simulink model "test_mdl"  (R2018a)
settings: Solver=VariableStepAuto  StartTime=0.0  StopTime=10.0  RelTol=1e-3
(part 3 of 8)

== system test_mdl/FD1_CAN_P702_GASD_MY21_DCV_V06/GWM/AC_Compressor_Data_FD1 ==
  ElCmprBattSysU_D_Falt : Constant
  ElCmprBattURng_D_Falt : Constant
  ElCmprInnrErr_D_Falt : Constant
  ElCmprLostComm_D_Falt : Constant
  ElCmprOverLoad_D_Falt : Constant
  ElCmprOverTe_D_Falt : Constant
  ElCmprOverTe_D_Stat : Constant
  ElCmprPerfErr_D_Falt : Constant
  ElCmprSysU_D_Falt : Constant
  ElCmprUHi_D_Stat : Constant
  ElCmprUHi_U_Actl : Constant
  ElCmpr_D_Stat : Constant
  ElCmpr_N_Actl : Constant
  ElCmpr_Pw_Actl : Constant
  bus_creator : BusCreator  Inputs=14
  port : Outport
  wires:
  bus_creator/1 -> port/1  "AC_Compressor_Data_FD1"
  ElCmprBattSysU_D_Falt/1 -> bus_creator/1  "ElCmprBattSysU_D_Falt"
  ElCmprBattURng_D_Falt/1 -> bus_creator/2  "ElCmprBattURng_D_Falt"
  ElCmprInnrErr_D_Falt/1 -> bus_creator/3  "ElCmprInnrErr_D_Falt"
  ElCmprLostComm_D_Falt/1 -> bus_creator/4  "ElCmprLostComm_D_Falt"
  ElCmprOverLoad_D_Falt/1 -> bus_creator/5  "ElCmprOverLoad_D_Falt"
  ElCmprOverTe_D_Falt/1 -> bus_creator/6  "ElCmprOverTe_D_Falt"
  ElCmprOverTe_D_Stat/1 -> bus_creator/7  "ElCmprOverTe_D_Stat"
  ElCmprPerfErr_D_Falt/1 -> bus_creator/8  "ElCmprPerfErr_D_Falt"
  ElCmprSysU_D_Falt/1 -> bus_creator/9  "ElCmprSysU_D_Falt"
  ElCmprUHi_D_Stat/1 -> bus_creator/10  "ElCmprUHi_D_Stat"
  ElCmprUHi_U_Actl/1 -> bus_creator/11  "ElCmprUHi_U_Actl"
  ElCmpr_D_Stat/1 -> bus_creator/12  "ElCmpr_D_Stat"
  ElCmpr_N_Actl/1 -> bus_creator/13  "ElCmpr_N_Actl"
  ElCmpr_Pw_Actl/1 -> bus_creator/14  "ElCmpr_Pw_Actl"

== system test_mdl/FD1_CAN_P702_GASD_MY21_DCV_V06/GWM/APIMGPS_Data_Nav_1_FD1 ==
  GPS_Latitude_Degrees : Constant
  GPS_Latitude_Min_dec : Constant
  GPS_Latitude_Minutes : Constant
  GPS_Longitude_Degrees : Constant
  GPS_Longitude_Min_dec : Constant
  GPS_Longitude_Minutes : Constant
  GpsHsphLattSth_D_Actl : Constant
  GpsHsphLongEast_D_Actl : Constant
  bus_creator : BusCreator  Inputs=8
  port : Outport
  wires:
  bus_creator/1 -> port/1  "APIMGPS_Data_Nav_1_FD1"
  GPS_Latitude_Degrees/1 -> bus_creator/1  "GPS_Latitude_Degrees"
  GPS_Latitude_Min_dec/1 -> bus_creator/2  "GPS_Latitude_Min_dec"
  GPS_Latitude_Minutes/1 -> bus_creator/3  "GPS_Latitude_Minutes"
  GPS_Longitude_Degrees/1 -> bus_creator/4  "GPS_Longitude_Degrees"
  GPS_Longitude_Min_dec/1 -> bus_creator/5  "GPS_Longitude_Min_dec"
  GPS_Longitude_Minutes/1 -> bus_creator/6  "GPS_Longitude_Minutes"
  GpsHsphLattSth_D_Actl/1 -> bus_creator/7  "GpsHsphLattSth_D_Actl"
  GpsHsphLongEast_D_Actl/1 -> bus_creator/8  "GpsHsphLongEast_D_Actl"

== system test_mdl/FD1_CAN_P702_GASD_MY21_DCV_V06/GWM/APIMGPS_Data_Nav_2_FD1 ==
  GPS_Actual_vs_Infer_pos : Constant
  GPS_Compass_direction : Constant
  GPS_Pdop : Constant
  GPS_UTC_hours : Constant
  GPS_UTC_minutes : Constant
  GPS_UTC_seconds : Constant
  GpsUtcDay_No_Actl : Constant
  GpsUtcMnth_No_Actl : Constant
  GpsUtcYr_No_Actl : Constant
  Gps_B_Falt : Constant
  bus_creator : BusCreator  Inputs=10
  port : Outport
  wires:
  bus_creator/1 -> port/1  "APIMGPS_Data_Nav_2_FD1"
  GPS_Actual_vs_Infer_pos/1 -> bus_creator/1  "GPS_Actual_vs_Infer_pos"
  GPS_Compass_direction/1 -> bus_creator/2  "GPS_Compass_direction"
  GPS_Pdop/1 -> bus_creator/3  "GPS_Pdop"
  GPS_UTC_hours/1 -> bus_creator/4  "GPS_UTC_hours"
  GPS_UTC_minutes/1 -> bus_creator/5  "GPS_UTC_minutes"
  GPS_UTC_seconds/1 -> bus_creator/6  "GPS_UTC_seconds"
  GpsUtcDay_No_Actl/1 -> bus_creator/7  "GpsUtcDay_No_Actl"
  GpsUtcMnth_No_Actl/1 -> bus_creator/8  "GpsUtcMnth_No_Actl"
  GpsUtcYr_No_Actl/1 -> bus_creator/9  "GpsUtcYr_No_Actl"
  Gps_B_Falt/1 -> bus_creator/10  "Gps_B_Falt"

== system test_mdl/FD1_CAN_P702_GASD_MY21_DCV_V06/GWM/APIMGPS_Data_Nav_3_FD1 ==
  GPS_Hdop : Constant
  GPS_Heading : Constant
  GPS_MSL_altitude : Constant
  GPS_Sat_num_in_view : Constant
  GPS_Speed : Constant
  GPS_Vdop : Constant
  GPS_dimension : Constant
  bus_creator : BusCreator  Inputs=7
  port : Outport
  wires:
  bus_creator/1 -> port/1  "APIMGPS_Data_Nav_3_FD1"
  GPS_Hdop/1 -> bus_creator/1  "GPS_Hdop"
  GPS_Heading/1 -> bus_creator/2  "GPS_Heading"
  GPS_MSL_altitude/1 -> bus_creator/3  "GPS_MSL_altitude"
  GPS_Sat_num_in_view/1 -> bus_creator/4  "GPS_Sat_num_in_view"
  GPS_Speed/1 -> bus_creator/5  "GPS_Speed"
  GPS_Vdop/1 -> bus_creator/6  "GPS_Vdop"
  GPS_dimension/1 -> bus_creator/7  "GPS_dimension"

== system test_mdl/FD1_CAN_P702_GASD_MY21_DCV_V06/GWM/APIM_Data_FD1 ==
  AutoLghtOvrrd_B_RqDrv : Constant
  DistToStopover_L_Actl : Constant
  ExtLghtDsply_D_Stat : Constant
  ExtLghtFront_D_RqMnu : Constant
  ExtLghtLeft_D_RqMnu : Constant
  ExtLghtRear_D_RqMnu : Constant
  ExtLghtRight_D_RqMnu : Constant
  GoTEditHr_T_RqMnu : Constant
  GoTEditMnte_T_RqMnu : Constant
  StopoverType_D_Stat : Constant
  bus_creator : BusCreator  Inputs=10
  port : Outport
  wires:
  bus_creator/1 -> port/1  "APIM_Data_FD1"
  AutoLghtOvrrd_B_RqDrv/1 -> bus_creator/1  "AutoLghtOvrrd_B_RqDrv"
  DistToStopover_L_Actl/1 -> bus_creator/2  "DistToStopover_L_Actl"
  ExtLghtDsply_D_Stat/1 -> bus_creator/3  "ExtLghtDsply_D_Stat"
  ExtLghtFront_D_RqMnu/1 -> bus_creator/4  "ExtLghtFront_D_RqMnu"
  ExtLghtLeft_D_RqMnu/1 -> bus_creator/5  "ExtLghtLeft_D_RqMnu"
  ExtLghtRear_D_RqMnu/1 -> bus_creator/6  "ExtLghtRear_D_RqMnu"
  ExtLghtRight_D_RqMnu/1 -> bus_creator/7  "ExtLghtRight_D_RqMnu"
  GoTEditHr_T_RqMnu/1 -> bus_creator/8  "GoTEditHr_T_RqMnu"
  GoTEditMnte_T_RqMnu/1 -> bus_creator/9  "GoTEditMnte_T_RqMnu"
  StopoverType_D_Stat/1 -> bus_creator/10  "StopoverType_D_Stat"

== system test_mdl/FD1_CAN_P702_GASD_MY21_DCV_V06/GWM/APIM_Request_Signals_1_FD1 ==
  Btt_L_Actl2 : Constant
  ChrgCrdLckEnbl_B_Stat : Constant
  ChrgOvrdExitScrn_D_Rq : Constant
  Cntr_Plg_Mode_Cmd : Constant
  EmPrflButtnAssoc_D_Rq : Constant
  EmPrflKeyAssoc_D_Rq : Constant
  EmPrflNo_D_Rq : Constant
  Em_D_Stat : Constant
  PmCabnLvl_D_Stat : Constant
  PmCabn_D_Stat : Constant
  PwRnngBoardMde_D_Rq : Constant
  PwRnngBoardSwtch_D_Rq : Constant
  PwRnngBoardT_D_Rq : Constant
  Rba_D_Rq : Constant
  bus_creator : BusCreator  Inputs=14
  port : Outport
  wires:
  bus_creator/1 -> port/1  "APIM_Request_Signals_1_FD1"
  Btt_L_Actl2/1 -> bus_creator/1  "Btt_L_Actl2"
  ChrgCrdLckEnbl_B_Stat/1 -> bus_creator/2  "ChrgCrdLckEnbl_B_Stat"
  ChrgOvrdExitScrn_D_Rq/1 -> bus_creator/3  "ChrgOvrdExitScrn_D_Rq"
  Cntr_Plg_Mode_Cmd/1 -> bus_creator/4  "Cntr_Plg_Mode_Cmd"
  EmPrflButtnAssoc_D_Rq/1 -> bus_creator/5  "EmPrflButtnAssoc_D_Rq"
  EmPrflKeyAssoc_D_Rq/1 -> bus_creator/6  "EmPrflKeyAssoc_D_Rq"
  EmPrflNo_D_Rq/1 -> bus_creator/7  "EmPrflNo_D_Rq"
  Em_D_Stat/1 -> bus_creator/8  "Em_D_Stat"
  PmCabnLvl_D_Stat/1 -> bus_creator/9  "PmCabnLvl_D_Stat"
  PmCabn_D_Stat/1 -> bus_creator/10  "PmCabn_D_Stat"
  PwRnngBoardMde_D_Rq/1 -> bus_creator/11  "PwRnngBoardMde_D_Rq"
  PwRnngBoardSwtch_D_Rq/1 -> bus_creator/12  "PwRnngBoardSwtch_D_Rq"
  PwRnngBoardT_D_Rq/1 -> bus_creator/13  "PwRnngBoardT_D_Rq"
  Rba_D_Rq/1 -> bus_creator/14  "Rba_D_Rq"

== system test_mdl/FD1_CAN_P702_GASD_MY21_DCV_V06/GWM/APIM_Request_Signals_5_FD1 ==
  OnbChrgLocIdTrgt_No_Rq : Constant
  OnbChrgLocIdUns_B_Rq : Constant
  OnbChrgPrflUpdate_B_Rq : Constant
  OnbChrgPrflWkdy_No_Rq : Constant
  OnbChrgPrflWknd_No_Rq : Constant
  OnbChrgSetDelete_B_Rq : Constant
  OnbChrgSetNow_D_Rq : Constant
  OnbChrgToPcWkdy_D_Actl : Constant
  OnbChrgToPcWknd_D_Actl : Constant
  bus_creator : BusCreator  Inputs=9
  port : Outport
  wires:
  bus_creator/1 -> port/1  "APIM_Request_Signals_5_FD1"
  OnbChrgLocIdTrgt_No_Rq/1 -> bus_creator/1  "OnbChrgLocIdTrgt_No_Rq"
  OnbChrgLocIdUns_B_Rq/1 -> bus_creator/2  "OnbChrgLocIdUns_B_Rq"
  OnbChrgPrflUpdate_B_Rq/1 -> bus_creator/3  "OnbChrgPrflUpdate_B_Rq"
  OnbChrgPrflWkdy_No_Rq/1 -> bus_creator/4  "OnbChrgPrflWkdy_No_Rq"
  OnbChrgPrflWknd_No_Rq/1 -> bus_creator/5  "OnbChrgPrflWknd_No_Rq"
  OnbChrgSetDelete_B_Rq/1 -> bus_creator/6  "OnbChrgSetDelete_B_Rq"
  OnbChrgSetNow_D_Rq/1 -> bus_creator/7  "OnbChrgSetNow_D_Rq"
  OnbChrgToPcWkdy_D_Actl/1 -> bus_creator/8  "OnbChrgToPcWkdy_D_Actl"
  OnbChrgToPcWknd_D_Actl/1 -> bus_creator/9  "OnbChrgToPcWknd_D_Actl"

== system test_mdl/FD1_CAN_P702_GASD_MY21_DCV_V06/GWM/APIM_Request_Signals_FD1 ==
  CbnCmrtPrefListIndx_Rq : Constant
  CbnCmrtPrefLstNmItm_Rq : Constant
  ChrgStatDsply_D_Rq : Constant
  FactoryReset_Rq : Constant
  LongTermParking_Rq : Constant
  ModemReset_D_Rq : Constant
  NextUsageTimeToggle_Rq : Constant
  OffPeakTimeSetHR_Rq : Constant
  OffPeakTimeSetMin_Rq : Constant
  StopStrtDrvMde_B_RqBtn3 : Constant
  TCU_ESN_D_Rq : Constant
  bus_creator : BusCreator  Inputs=11
  port : Outport
  wires:
  bus_creator/1 -> port/1  "APIM_Request_Signals_FD1"
  CbnCmrtPrefListIndx_Rq/1 -> bus_creator/1  "CbnCmrtPrefListIndx_Rq"
  CbnCmrtPrefLstNmItm_Rq/1 -> bus_creator/2  "CbnCmrtPrefLstNmItm_Rq"
  ChrgStatDsply_D_Rq/1 -> bus_creator/3  "ChrgStatDsply_D_Rq"
  FactoryReset_Rq/1 -> bus_creator/4  "FactoryReset_Rq"
  LongTermParking_Rq/1 -> bus_creator/5  "LongTermParking_Rq"
  ModemReset_D_Rq/1 -> bus_creator/6  "ModemReset_D_Rq"
  NextUsageTimeToggle_Rq/1 -> bus_creator/7  "NextUsageTimeToggle_Rq"
  OffPeakTimeSetHR_Rq/1 -> bus_creator/8  "OffPeakTimeSetHR_Rq"
  OffPeakTimeSetMin_Rq/1 -> bus_creator/9  "OffPeakTimeSetMin_Rq"
  StopStrtDrvMde_B_RqBtn3/1 -> bus_creator/10  "StopStrtDrvMde_B_RqBtn3"
  TCU_ESN_D_Rq/1 -> bus_creator/11  "TCU_ESN_D_Rq"

== system test_mdl/FD1_CAN_P702_GASD_MY21_DCV_V06/GWM/APIM_Send_Signals1_FD1 ==
  APIM_ActiveTrackNum_St : Constant
  APIM_NumberofTracks_St : Constant
  AutoHoldSwtch_D_Stat3 : Constant
  CenterStackRing_D_Actl : Constant
  ChrgCordUnlock_B_Rq : Constant
  TrlrAidCancl_B_Rq : Constant
  TrlrAidSetup_D_Stat : Constant
  TrlrTrgtAcquire_D_Rq : Constant
  ValetMode_D_Stat : Constant
  bus_creator : BusCreator  Inputs=9
  port : Outport
  wires:
  bus_creator/1 -> port/1  "APIM_Send_Signals1_FD1"
  APIM_ActiveTrackNum_St/1 -> bus_creator/1  "APIM_ActiveTrackNum_St"
  APIM_NumberofTracks_St/1 -> bus_creator/2  "APIM_NumberofTracks_St"
  AutoHoldSwtch_D_Stat3/1 -> bus_creator/3  "AutoHoldSwtch_D_Stat3"
  CenterStackRing_D_Actl/1 -> bus_creator/4  "CenterStackRing_D_Actl"
  ChrgCordUnlock_B_Rq/1 -> bus_creator/5  "ChrgCordUnlock_B_Rq"
  TrlrAidCancl_B_Rq/1 -> bus_creator/6  "TrlrAidCancl_B_Rq"
  TrlrAidSetup_D_Stat/1 -> bus_creator/7  "TrlrAidSetup_D_Stat"
  TrlrTrgtAcquire_D_Rq/1 -> bus_creator/8  "TrlrTrgtAcquire_D_Rq"
  ValetMode_D_Stat/1 -> bus_creator/9  "ValetMode_D_Stat"

== system test_mdl/FD1_CAN_P702_GASD_MY21_DCV_V06/GWM/APIM_Send_Signals_2_FD1 ==
  AutoEpbButtn_B_Stat : Constant
  AutoEpbZoomView_B_Stat : Constant
  DcacGfciTestBttn_B_Stat : Constant
  DcacPwButtn_B_Falt : Constant
  DcacPwHiButtn_B_Stat : Constant
  DcacPwLoButtn_B_Stat : Constant
  DcacPwOffButtn_B_Stat : Constant
  DcacPwResetButtn_B_Stat : Constant
  OnbChrgClearAll_B_Rq : Constant
  OnbChrgGoTDelete_B_Rq : Constant
  OnbChrgGoTElement_D_Rq : Constant
  OnbChrgGoTExtHtr_D_Rq : Constant
  OnbChrgGoTHr_T_Rq : Constant
  OnbChrgGoTMnte_D_Rq : Constant
  OnbChrgGoTOn_D_Rq : Constant
  OnbChrgGoTPrcond_D_Rq : Constant
  OnbChrgGoTTouch_D_Rq : Constant
  OnbChrgGoTUpdate_B_Rq : Constant
  OtaTrg_D_Stat : Constant
  PaakMyKey_D_Rq : Constant
  TCU_Final_Actvtn_St : Constant
  TCU_Init_Actvtn_St : Constant
  TrlrAidMde_D_Rq : Constant
  TrlrBrkGain_No_Rq : Constant
  TrlrHitch_D_RqMnu : Constant
  bus_creator : BusCreator  Inputs=25
  port : Outport
  wires:
  bus_creator/1 -> port/1  "APIM_Send_Signals_2_FD1"
  AutoEpbButtn_B_Stat/1 -> bus_creator/1  "AutoEpbButtn_B_Stat"
  AutoEpbZoomView_B_Stat/1 -> bus_creator/2  "AutoEpbZoomView_B_Stat"
  DcacGfciTestBttn_B_Stat/1 -> bus_creator/3  "DcacGfciTestBttn_B_Stat"
  DcacPwButtn_B_Falt/1 -> bus_creator/4  "DcacPwButtn_B_Falt"
  DcacPwHiButtn_B_Stat/1 -> bus_creator/5  "DcacPwHiButtn_B_Stat"
  DcacPwLoButtn_B_Stat/1 -> bus_creator/6  "DcacPwLoButtn_B_Stat"
  DcacPwOffButtn_B_Stat/1 -> bus_creator/7  "DcacPwOffButtn_B_Stat"
  DcacPwResetButtn_B_Stat/1 -> bus_creator/8  "DcacPwResetButtn_B_Stat"
  OnbChrgClearAll_B_Rq/1 -> bus_creator/9  "OnbChrgClearAll_B_Rq"
  OnbChrgGoTDelete_B_Rq/1 -> bus_creator/10  "OnbChrgGoTDelete_B_Rq"
  OnbChrgGoTElement_D_Rq/1 -> bus_creator/11  "OnbChrgGoTElement_D_Rq"
  OnbChrgGoTExtHtr_D_Rq/1 -> bus_creator/12  "OnbChrgGoTExtHtr_D_Rq"
  OnbChrgGoTHr_T_Rq/1 -> bus_creator/13  "OnbChrgGoTHr_T_Rq"
  OnbChrgGoTMnte_D_Rq/1 -> bus_creator/14  "OnbChrgGoTMnte_D_Rq"
  OnbChrgGoTOn_D_Rq/1 -> bus_creator/15  "OnbChrgGoTOn_D_Rq"
  OnbChrgGoTPrcond_D_Rq/1 -> bus_creator/16  "OnbChrgGoTPrcond_D_Rq"
  OnbChrgGoTTouch_D_Rq/1 -> bus_creator/17  "OnbChrgGoTTouch_D_Rq"
  OnbChrgGoTUpdate_B_Rq/1 -> bus_creator/18  "OnbChrgGoTUpdate_B_Rq"
  OtaTrg_D_Stat/1 -> bus_creator/19  "OtaTrg_D_Stat"
  PaakMyKey_D_Rq/1 -> bus_creator/20  "PaakMyKey_D_Rq"
  TCU_Final_Actvtn_St/1 -> bus_creator/21  "TCU_Final_Actvtn_St"
  TCU_Init_Actvtn_St/1 -> bus_creator/22  "TCU_Init_Actvtn_St"
  TrlrAidMde_D_Rq/1 -> bus_creator/23  "TrlrAidMde_D_Rq"
  TrlrBrkGain_No_Rq/1 -> bus_creator/24  "TrlrBrkGain_No_Rq"
  TrlrHitch_D_RqMnu/1 -> bus_creator/25  "TrlrHitch_D_RqMnu"

== system test_mdl/FD1_CAN_P702_GASD_MY21_DCV_V06/GWM/Accel_Data_FD1 ==
  VehLat2_A_Actl : Constant
  VehLatAActl_D_Qf : Constant
  VehLatLongVertA_No_Cs : Constant
  VehLatLongVert_No_Cnt : Constant
  VehLong2_A_Actl : Constant
  VehLongAActl_D_Qf : Constant
  VehVert2_A_Actl : Constant
  VehVertAActl_D_Qf : Constant
  bus_creator : BusCreator  Inputs=8
  port : Outport
  wires:
  bus_creator/1 -> port/1  "Accel_Data_FD1"
  VehLat2_A_Actl/1 -> bus_creator/1  "VehLat2_A_Actl"
  VehLatAActl_D_Qf/1 -> bus_creator/2  "VehLatAActl_D_Qf"
  VehLatLongVertA_No_Cs/1 -> bus_creator/3  "VehLatLongVertA_No_Cs"
  VehLatLongVert_No_Cnt/1 -> bus_creator/4  "VehLatLongVert_No_Cnt"
  VehLong2_A_Actl/1 -> bus_creator/5  "VehLong2_A_Actl"
  VehLongAActl_D_Qf/1 -> bus_creator/6  "VehLongAActl_D_Qf"
  VehVert2_A_Actl/1 -> bus_creator/7  "VehVert2_A_Actl"
  VehVertAActl_D_Qf/1 -> bus_creator/8  "VehVertAActl_D_Qf"

== system test_mdl/FD1_CAN_P702_GASD_MY21_DCV_V06/GWM/ActiveFrontStrg_Stat2_FD1 ==
  SteWhlRelCalib_An_Sns : Constant
  SteWhlRelCalib_T_Actl : Constant
  bus_creator : BusCreator  Inputs=2
  port : Outport
  wires:
  bus_creator/1 -> port/1  "ActiveFrontStrg_Stat2_FD1"
  SteWhlRelCalib_An_Sns/1 -> bus_creator/1  "SteWhlRelCalib_An_Sns"
  SteWhlRelCalib_T_Actl/1 -> bus_creator/2  "SteWhlRelCalib_T_Actl"

== system test_mdl/FD1_CAN_P702_GASD_MY21_DCV_V06/GWM/ActiveFrontStrg_Stat_FD1 ==
  SteWhlBrkAnActl_No_Cnt : Constant
  SteWhlBrkAnActl_No_Cs : Constant
  SteWhlBrkOffst_An_Actl : Constant
  SteWhlOffstRq_D_Stat : Constant
  SteWhlOffst_An_TotActl : Constant
  bus_creator : BusCreator  Inputs=5
  port : Outport
  wires:
  bus_creator/1 -> port/1  "ActiveFrontStrg_Stat_FD1"
  SteWhlBrkAnActl_No_Cnt/1 -> bus_creator/1  "SteWhlBrkAnActl_No_Cnt"
  SteWhlBrkAnActl_No_Cs/1 -> bus_creator/2  "SteWhlBrkAnActl_No_Cs"
  SteWhlBrkOffst_An_Actl/1 -> bus_creator/3  "SteWhlBrkOffst_An_Actl"
  SteWhlOffstRq_D_Stat/1 -> bus_creator/4  "SteWhlOffstRq_D_Stat"
  SteWhlOffst_An_TotActl/1 -> bus_creator/5  "SteWhlOffst_An_TotActl"

== system test_mdl/FD1_CAN_P702_GASD_MY21_DCV_V06/GWM/Adaptive_Headlamp_Stat ==
  Adaptive_Hdlmp_Fault : Constant
  AhbStatGfhbFdbk_D_Actl : Constant
  HeadLghtDrvSide_B_Stat : Constant
  HeadLghtHiOn_B_StatHcm : Constant
  bus_creator : BusCreator  Inputs=4
  port : Outport
  wires:
  bus_creator/1 -> port/1  "Adaptive_Headlamp_Stat"
  Adaptive_Hdlmp_Fault/1 -> bus_creator/1  "Adaptive_Hdlmp_Fault"
  AhbStatGfhbFdbk_D_Actl/1 -> bus_creator/2  "AhbStatGfhbFdbk_D_Actl"
  HeadLghtDrvSide_B_Stat/1 -> bus_creator/3  "HeadLghtDrvSide_B_Stat"
  HeadLghtHiOn_B_StatHcm/1 -> bus_creator/4  "HeadLghtHiOn_B_StatHcm"

== system test_mdl/FD1_CAN_P702_GASD_MY21_DCV_V06/GWM/AllTerrainControlData_FD1 ==
  SelDrvMdeCnt_D_Stat : Constant
  SelDrvMdeSwtch_D_Stat : Constant
  SelDrvMdeSwtch_No_Actl : Constant
  bus_creator : BusCreator  Inputs=3
  port : Outport
  wires:
  bus_creator/1 -> port/1  "AllTerrainControlData_FD1"
  SelDrvMdeCnt_D_Stat/1 -> bus_creator/1  "SelDrvMdeCnt_D_Stat"
  SelDrvMdeSwtch_D_Stat/1 -> bus_creator/2  "SelDrvMdeSwtch_D_Stat"
  SelDrvMdeSwtch_No_Actl/1 -> bus_creator/3  "SelDrvMdeSwtch_No_Actl"

== system test_mdl/FD1_CAN_P702_GASD_MY21_DCV_V06/GWM/All_Terrain_Data_FD1 ==
  TerrMde_D_RqDrv : Constant
  bus_creator : BusCreator  Inputs=1
  port : Outport
  wires:
  bus_creator/1 -> port/1  "All_Terrain_Data_FD1"
  TerrMde_D_RqDrv/1 -> bus_creator/1  "TerrMde_D_RqDrv"

== system test_mdl/FD1_CAN_P702_GASD_MY21_DCV_V06/GWM/BCMC_Data_FD1 ==
  WndwRearHeat_D_Stat : Constant
  WndwRearHeat_I_Actl : Constant
  bus_creator : BusCreator  Inputs=2
  port : Outport
  wires:
  bus_creator/1 -> port/1  "BCMC_Data_FD1"
  WndwRearHeat_D_Stat/1 -> bus_creator/1  "WndwRearHeat_D_Stat"
  WndwRearHeat_I_Actl/1 -> bus_creator/2  "WndwRearHeat_I_Actl"

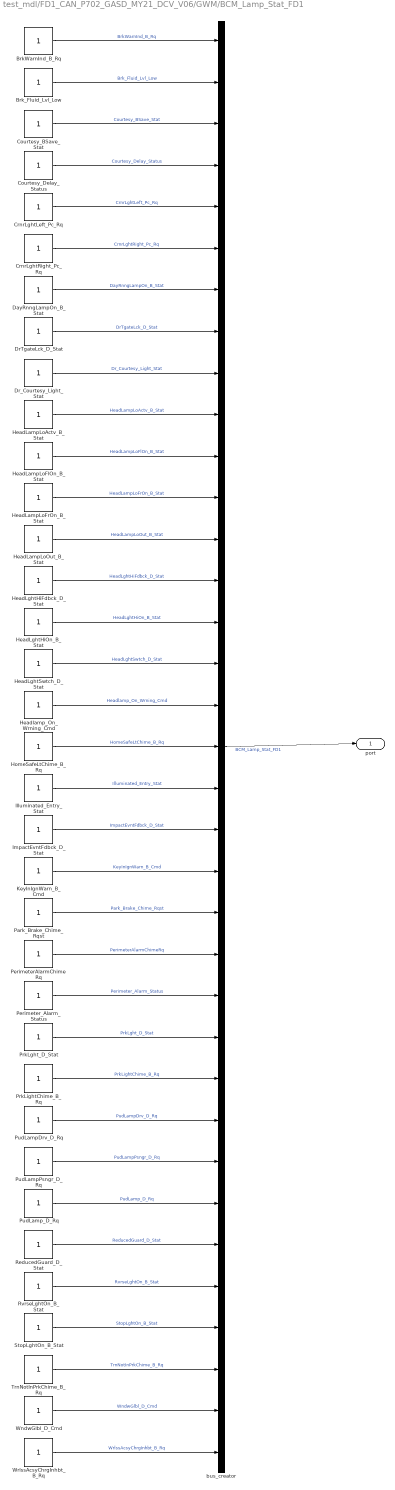
== system test_mdl/FD1_CAN_P702_GASD_MY21_DCV_V06/GWM/BCM_Lamp_Stat_FD1 ==
  BrkWarnInd_B_Rq : Constant
  Brk_Fluid_Lvl_Low : Constant
  Courtesy_BSave_Stat : Constant
  Courtesy_Delay_Status : Constant
  CrnrLghtLeft_Pc_Rq : Constant
  CrnrLghtRight_Pc_Rq : Constant
  DayRnngLampOn_B_Stat : Constant
  DrTgateLck_D_Stat : Constant
  Dr_Courtesy_Light_Stat : Constant
  HeadLampLoActv_B_Stat : Constant
  HeadLampLoFlOn_B_Stat : Constant
  HeadLampLoFrOn_B_Stat : Constant
  HeadLampLoOut_B_Stat : Constant
  HeadLghtHiFdbck_D_Stat : Constant
  HeadLghtHiOn_B_Stat : Constant
  HeadLghtSwtch_D_Stat : Constant
  Headlamp_On_Wrning_Cmd : Constant
  HomeSafeLtChime_B_Rq : Constant
  Illuminated_Entry_Stat : Constant
  ImpactEvntFdbck_D_Stat : Constant
  KeyInIgnWarn_B_Cmd : Constant
  Park_Brake_Chime_Rqst : Constant
  PerimeterAlarmChimeRq : Constant
  Perimeter_Alarm_Status : Constant
  PrkLght_D_Stat : Constant
  PrkLightChime_B_Rq : Constant
  PudLampDrv_D_Rq : Constant
  PudLampPsngr_D_Rq : Constant
  PudLamp_D_Rq : Constant
  ReducedGuard_D_Stat : Constant
  RvrseLghtOn_B_Stat : Constant
  StopLghtOn_B_Stat : Constant
  TrnNotInPrkChime_B_Rq : Constant
  WndwGlbl_D_Cmd : Constant
  WrlssAcsyChrgInhbt_B_Rq : Constant
  bus_creator : BusCreator  Inputs=35
  port : Outport
  wires:
  bus_creator/1 -> port/1  "BCM_Lamp_Stat_FD1"
  BrkWarnInd_B_Rq/1 -> bus_creator/1  "BrkWarnInd_B_Rq"
  Brk_Fluid_Lvl_Low/1 -> bus_creator/2  "Brk_Fluid_Lvl_Low"
  Courtesy_BSave_Stat/1 -> bus_creator/3  "Courtesy_BSave_Stat"
  Courtesy_Delay_Status/1 -> bus_creator/4  "Courtesy_Delay_Status"
  CrnrLghtLeft_Pc_Rq/1 -> bus_creator/5  "CrnrLghtLeft_Pc_Rq"
  CrnrLghtRight_Pc_Rq/1 -> bus_creator/6  "CrnrLghtRight_Pc_Rq"
  DayRnngLampOn_B_Stat/1 -> bus_creator/7  "DayRnngLampOn_B_Stat"
  DrTgateLck_D_Stat/1 -> bus_creator/8  "DrTgateLck_D_Stat"
  Dr_Courtesy_Light_Stat/1 -> bus_creator/9  "Dr_Courtesy_Light_Stat"
  HeadLampLoActv_B_Stat/1 -> bus_creator/10  "HeadLampLoActv_B_Stat"
  HeadLampLoFlOn_B_Stat/1 -> bus_creator/11  "HeadLampLoFlOn_B_Stat"
  HeadLampLoFrOn_B_Stat/1 -> bus_creator/12  "HeadLampLoFrOn_B_Stat"
  HeadLampLoOut_B_Stat/1 -> bus_creator/13  "HeadLampLoOut_B_Stat"
  HeadLghtHiFdbck_D_Stat/1 -> bus_creator/14  "HeadLghtHiFdbck_D_Stat"
  HeadLghtHiOn_B_Stat/1 -> bus_creator/15  "HeadLghtHiOn_B_Stat"
  HeadLghtSwtch_D_Stat/1 -> bus_creator/16  "HeadLghtSwtch_D_Stat"
  Headlamp_On_Wrning_Cmd/1 -> bus_creator/17  "Headlamp_On_Wrning_Cmd"
  HomeSafeLtChime_B_Rq/1 -> bus_creator/18  "HomeSafeLtChime_B_Rq"
  Illuminated_Entry_Stat/1 -> bus_creator/19  "Illuminated_Entry_Stat"
  ImpactEvntFdbck_D_Stat/1 -> bus_creator/20  "ImpactEvntFdbck_D_Stat"
  KeyInIgnWarn_B_Cmd/1 -> bus_creator/21  "KeyInIgnWarn_B_Cmd"
  Park_Brake_Chime_Rqst/1 -> bus_creator/22  "Park_Brake_Chime_Rqst"
  PerimeterAlarmChimeRq/1 -> bus_creator/23  "PerimeterAlarmChimeRq"
  Perimeter_Alarm_Status/1 -> bus_creator/24  "Perimeter_Alarm_Status"
  PrkLght_D_Stat/1 -> bus_creator/25  "PrkLght_D_Stat"
  PrkLightChime_B_Rq/1 -> bus_creator/26  "PrkLightChime_B_Rq"
  PudLampDrv_D_Rq/1 -> bus_creator/27  "PudLampDrv_D_Rq"
  PudLampPsngr_D_Rq/1 -> bus_creator/28  "PudLampPsngr_D_Rq"
  PudLamp_D_Rq/1 -> bus_creator/29  "PudLamp_D_Rq"
  ReducedGuard_D_Stat/1 -> bus_creator/30  "ReducedGuard_D_Stat"
  RvrseLghtOn_B_Stat/1 -> bus_creator/31  "RvrseLghtOn_B_Stat"
  StopLghtOn_B_Stat/1 -> bus_creator/32  "StopLghtOn_B_Stat"
  TrnNotInPrkChime_B_Rq/1 -> bus_creator/33  "TrnNotInPrkChime_B_Rq"
  WndwGlbl_D_Cmd/1 -> bus_creator/34  "WndwGlbl_D_Cmd"
  WrlssAcsyChrgInhbt_B_Rq/1 -> bus_creator/35  "WrlssAcsyChrgInhbt_B_Rq"

== system test_mdl/FD1_CAN_P702_GASD_MY21_DCV_V06/GWM/BattRgenLo_1_FD1 ==
  BattRgenLo_I_Actl : Constant
  BattRgenLo_U_Actl : Constant
  bus_creator : BusCreator  Inputs=2
  port : Outport
  wires:
  bus_creator/1 -> port/1  "BattRgenLo_1_FD1"
  BattRgenLo_I_Actl/1 -> bus_creator/1  "BattRgenLo_I_Actl"
  BattRgenLo_U_Actl/1 -> bus_creator/2  "BattRgenLo_U_Actl"

== system test_mdl/FD1_CAN_P702_GASD_MY21_DCV_V06/GWM/BattRgenLo_2_FD1 ==
  BattRgenLoChrg_I_Mx : Constant
  BattRgenLoChrg_U_Mx : Constant
  BattRgenLoDchrg_I_Mx : Constant
  BattRgenLoDchrg_U_Mn : Constant
  BattRgenLoOpen_U_Actl : Constant
  bus_creator : BusCreator  Inputs=5
  port : Outport
  wires:
  bus_creator/1 -> port/1  "BattRgenLo_2_FD1"
  BattRgenLoChrg_I_Mx/1 -> bus_creator/1  "BattRgenLoChrg_I_Mx"
  BattRgenLoChrg_U_Mx/1 -> bus_creator/2  "BattRgenLoChrg_U_Mx"
  BattRgenLoDchrg_I_Mx/1 -> bus_creator/3  "BattRgenLoDchrg_I_Mx"
  BattRgenLoDchrg_U_Mn/1 -> bus_creator/4  "BattRgenLoDchrg_U_Mn"
  BattRgenLoOpen_U_Actl/1 -> bus_creator/5  "BattRgenLoOpen_U_Actl"

== system test_mdl/FD1_CAN_P702_GASD_MY21_DCV_V06/GWM/BattRgenLo_3_FD1 ==
  BattRgenLoBalnc_B_Rq : Constant
  BattRgenLo_AhRide_Actl : Constant
  BattRgenLo_Ah_Actl : Constant
  BattRgenLo_R_Actl : Constant
  BattRgenLo_Te_Actl : Constant
  BattRgenLo_Te_Hi : Constant
  bus_creator : BusCreator  Inputs=6
  port : Outport
  wires:
  bus_creator/1 -> port/1  "BattRgenLo_3_FD1"
  BattRgenLoBalnc_B_Rq/1 -> bus_creator/1  "BattRgenLoBalnc_B_Rq"
  BattRgenLo_AhRide_Actl/1 -> bus_creator/2  "BattRgenLo_AhRide_Actl"
  BattRgenLo_Ah_Actl/1 -> bus_creator/3  "BattRgenLo_Ah_Actl"
  BattRgenLo_R_Actl/1 -> bus_creator/4  "BattRgenLo_R_Actl"
  BattRgenLo_Te_Actl/1 -> bus_creator/5  "BattRgenLo_Te_Actl"
  BattRgenLo_Te_Hi/1 -> bus_creator/6  "BattRgenLo_Te_Hi"

== system test_mdl/FD1_CAN_P702_GASD_MY21_DCV_V06/GWM/BattRgenLo_4_FD1 ==
  BattRgenLoChrg_B_Rq : Constant
  BattRgenLoChrg_D_Stat : Constant
  BattRgenLoDChrg_D_Stat : Constant
  BattRgenLoDchrg_B_Rq : Constant
  BattRgenLoPrtct_B_Stat : Constant
  BattRgenLoPulse_U_Pred : Constant
  BattRgenLoSoc_Pc_Actl : Constant
  BattRgenLoStat_D_Qlty : Constant
  BattRgenLo_B_Falt : Constant
  BattRgenLo_T_Est : Constant
  bus_creator : BusCreator  Inputs=10
  port : Outport
  wires:
  bus_creator/1 -> port/1  "BattRgenLo_4_FD1"
  BattRgenLoChrg_B_Rq/1 -> bus_creator/1  "BattRgenLoChrg_B_Rq"
  BattRgenLoChrg_D_Stat/1 -> bus_creator/2  "BattRgenLoChrg_D_Stat"
  BattRgenLoDChrg_D_Stat/1 -> bus_creator/3  "BattRgenLoDChrg_D_Stat"
  BattRgenLoDchrg_B_Rq/1 -> bus_creator/4  "BattRgenLoDchrg_B_Rq"
  BattRgenLoPrtct_B_Stat/1 -> bus_creator/5  "BattRgenLoPrtct_B_Stat"
  BattRgenLoPulse_U_Pred/1 -> bus_creator/6  "BattRgenLoPulse_U_Pred"
  BattRgenLoSoc_Pc_Actl/1 -> bus_creator/7  "BattRgenLoSoc_Pc_Actl"
  BattRgenLoStat_D_Qlty/1 -> bus_creator/8  "BattRgenLoStat_D_Qlty"
  BattRgenLo_B_Falt/1 -> bus_creator/9  "BattRgenLo_B_Falt"
  BattRgenLo_T_Est/1 -> bus_creator/10  "BattRgenLo_T_Est"

== system test_mdl/FD1_CAN_P702_GASD_MY21_DCV_V06/GWM/Battery_Mgmt_24V_FD1 ==
  BattULo24Soc_Pc_Actl : Constant
  BattULo24State_D_Qlty : Constant
  BattULo24_Ah_DeltaRide : Constant
  BattULo24_B_Falt : Constant
  BattULo24_D_Falt : Constant
  BattULo24_I_Actl : Constant
  BattULo24_Te_Actl : Constant
  bus_creator : BusCreator  Inputs=7
  port : Outport
  wires:
  bus_creator/1 -> port/1  "Battery_Mgmt_24V_FD1"
  BattULo24Soc_Pc_Actl/1 -> bus_creator/1  "BattULo24Soc_Pc_Actl"
  BattULo24State_D_Qlty/1 -> bus_creator/2  "BattULo24State_D_Qlty"
  BattULo24_Ah_DeltaRide/1 -> bus_creator/3  "BattULo24_Ah_DeltaRide"
  BattULo24_B_Falt/1 -> bus_creator/4  "BattULo24_B_Falt"
  BattULo24_D_Falt/1 -> bus_creator/5  "BattULo24_D_Falt"
  BattULo24_I_Actl/1 -> bus_creator/6  "BattULo24_I_Actl"
  BattULo24_Te_Actl/1 -> bus_creator/7  "BattULo24_Te_Actl"

== system test_mdl/FD1_CAN_P702_GASD_MY21_DCV_V06/GWM/Battery_Mgmt_2_FD1 ==
  BattULoChrg_D_Rq : Constant
  BattULoSrvc_T_Actl : Constant
  Batt_Crit_SoC_B : Constant
  Batt_Lo_SoC_B : Constant
  ChargeMode : Constant
  EngStrtInhbt_B_RqBatt : Constant
  IdleSpeedIncrease_El : Constant
  PeriodicElLoad_B_Stat : Constant
  PwSysULoFalt_D_Stat : Constant
  Shed_Drain_Eng_Off_B : Constant
  Shed_Feature_Group_ID : Constant
  Shed_Level_Req : Constant
  Shed_T_Eng_Off_B : Constant
  ULoRgenTestMde_B_Rq : Constant
  bus_creator : BusCreator  Inputs=14
  port : Outport
  wires:
  bus_creator/1 -> port/1  "Battery_Mgmt_2_FD1"
  BattULoChrg_D_Rq/1 -> bus_creator/1  "BattULoChrg_D_Rq"
  BattULoSrvc_T_Actl/1 -> bus_creator/2  "BattULoSrvc_T_Actl"
  Batt_Crit_SoC_B/1 -> bus_creator/3  "Batt_Crit_SoC_B"
  Batt_Lo_SoC_B/1 -> bus_creator/4  "Batt_Lo_SoC_B"
  ChargeMode/1 -> bus_creator/5  "ChargeMode"
  EngStrtInhbt_B_RqBatt/1 -> bus_creator/6  "EngStrtInhbt_B_RqBatt"
  IdleSpeedIncrease_El/1 -> bus_creator/7  "IdleSpeedIncrease_El"
  PeriodicElLoad_B_Stat/1 -> bus_creator/8  "PeriodicElLoad_B_Stat"
  PwSysULoFalt_D_Stat/1 -> bus_creator/9  "PwSysULoFalt_D_Stat"
  Shed_Drain_Eng_Off_B/1 -> bus_creator/10  "Shed_Drain_Eng_Off_B"
  Shed_Feature_Group_ID/1 -> bus_creator/11  "Shed_Feature_Group_ID"
  Shed_Level_Req/1 -> bus_creator/12  "Shed_Level_Req"
  Shed_T_Eng_Off_B/1 -> bus_creator/13  "Shed_T_Eng_Off_B"
  ULoRgenTestMde_B_Rq/1 -> bus_creator/14  "ULoRgenTestMde_B_Rq"

== system test_mdl/FD1_CAN_P702_GASD_MY21_DCV_V06/GWM/Battery_Mgmt_3_FD1 ==
  BSBattQCapAh : Constant
  BSBattQDeltaRideAh : Constant
  BSBattSOC : Constant
  BSFault : Constant
  BattULo2_Te_Actl : Constant
  BattULoChrg_URate_RqMx : Constant
  BattULoChrg_U_RqMn : Constant
  BattULoChrg_U_RqMx : Constant
  BattULoState_D_Qlty : Constant
  bus_creator : BusCreator  Inputs=9
  port : Outport
  wires:
  bus_creator/1 -> port/1  "Battery_Mgmt_3_FD1"
  BSBattQCapAh/1 -> bus_creator/1  "BSBattQCapAh"
  BSBattQDeltaRideAh/1 -> bus_creator/2  "BSBattQDeltaRideAh"
  BSBattSOC/1 -> bus_creator/3  "BSBattSOC"
  BSFault/1 -> bus_creator/4  "BSFault"
  BattULo2_Te_Actl/1 -> bus_creator/5  "BattULo2_Te_Actl"
  BattULoChrg_URate_RqMx/1 -> bus_creator/6  "BattULoChrg_URate_RqMx"
  BattULoChrg_U_RqMn/1 -> bus_creator/7  "BattULoChrg_U_RqMn"
  BattULoChrg_U_RqMx/1 -> bus_creator/8  "BattULoChrg_U_RqMx"
  BattULoState_D_Qlty/1 -> bus_creator/9  "BattULoState_D_Qlty"

== system test_mdl/FD1_CAN_P702_GASD_MY21_DCV_V06/GWM/Battery_Mgmt_4_FD1 ==
  BattULoAuxIsol_D_Rq : Constant
  BattULoAuxSoc_Pc_Actl : Constant
  BattULoAux_B_Falt : Constant
  BattULoAux_D_Qlty : Constant
  BattULoAux_I_Actl : Constant
  BattULoAux_U_Actl : Constant
  BattULoAux_U_Rq : Constant
  BattULoCrnkBelt_U_Pred : Constant
  BattULoCrnkStrt_U_Pred : Constant
  bus_creator : BusCreator  Inputs=9
  port : Outport
  wires:
  bus_creator/1 -> port/1  "Battery_Mgmt_4_FD1"
  BattULoAuxIsol_D_Rq/1 -> bus_creator/1  "BattULoAuxIsol_D_Rq"
  BattULoAuxSoc_Pc_Actl/1 -> bus_creator/2  "BattULoAuxSoc_Pc_Actl"
  BattULoAux_B_Falt/1 -> bus_creator/3  "BattULoAux_B_Falt"
  BattULoAux_D_Qlty/1 -> bus_creator/4  "BattULoAux_D_Qlty"
  BattULoAux_I_Actl/1 -> bus_creator/5  "BattULoAux_I_Actl"
  BattULoAux_U_Actl/1 -> bus_creator/6  "BattULoAux_U_Actl"
  BattULoAux_U_Rq/1 -> bus_creator/7  "BattULoAux_U_Rq"
  BattULoCrnkBelt_U_Pred/1 -> bus_creator/8  "BattULoCrnkBelt_U_Pred"
  BattULoCrnkStrt_U_Pred/1 -> bus_creator/9  "BattULoCrnkStrt_U_Pred"

== system test_mdl/FD1_CAN_P702_GASD_MY21_DCV_V06/GWM/Battery_Traction_1_FD1 ==
  BattTracMil_D_Rq : Constant
  BattTracOffFst_D_Actl : Constant
  BattTracOff_B_Actl : Constant
  BattTrac_I_Actl : Constant
  BattTrac_U_Actl : Constant
  BattTrac_U_LimHi : Constant
  BattTrac_U_LimLo : Constant
  VehStrtInhbt_B_RqBatt : Constant
  bus_creator : BusCreator  Inputs=8
  port : Outport
  wires:
  bus_creator/1 -> port/1  "Battery_Traction_1_FD1"
  BattTracMil_D_Rq/1 -> bus_creator/1  "BattTracMil_D_Rq"
  BattTracOffFst_D_Actl/1 -> bus_creator/2  "BattTracOffFst_D_Actl"
  BattTracOff_B_Actl/1 -> bus_creator/3  "BattTracOff_B_Actl"
  BattTrac_I_Actl/1 -> bus_creator/4  "BattTrac_I_Actl"
  BattTrac_U_Actl/1 -> bus_creator/5  "BattTrac_U_Actl"
  BattTrac_U_LimHi/1 -> bus_creator/6  "BattTrac_U_LimHi"
  BattTrac_U_LimLo/1 -> bus_creator/7  "BattTrac_U_LimLo"
  VehStrtInhbt_B_RqBatt/1 -> bus_creator/8  "VehStrtInhbt_B_RqBatt"

== system test_mdl/FD1_CAN_P702_GASD_MY21_DCV_V06/GWM/Battery_Traction_3_FD1 ==
  BattTracClnt_Te_Actl : Constant
  BattTracSoc_Pc_LimHi : Constant
  BattTracSoc_Pc_LimLo : Constant
  BattTracSoc_Pc_MnPrtct : Constant
  BattTracSoc_Pc_MxPrtct : Constant
  BattTracSrvcRqd_B_Rq : Constant
  BattTracWarnLamp_B_Rq : Constant
  bus_creator : BusCreator  Inputs=7
  port : Outport
  wires:
  bus_creator/1 -> port/1  "Battery_Traction_3_FD1"
  BattTracClnt_Te_Actl/1 -> bus_creator/1  "BattTracClnt_Te_Actl"
  BattTracSoc_Pc_LimHi/1 -> bus_creator/2  "BattTracSoc_Pc_LimHi"
  BattTracSoc_Pc_LimLo/1 -> bus_creator/3  "BattTracSoc_Pc_LimLo"
  BattTracSoc_Pc_MnPrtct/1 -> bus_creator/4  "BattTracSoc_Pc_MnPrtct"
  BattTracSoc_Pc_MxPrtct/1 -> bus_creator/5  "BattTracSoc_Pc_MxPrtct"
  BattTracSrvcRqd_B_Rq/1 -> bus_creator/6  "BattTracSrvcRqd_B_Rq"
  BattTracWarnLamp_B_Rq/1 -> bus_creator/7  "BattTracWarnLamp_B_Rq"

== system test_mdl/FD1_CAN_P702_GASD_MY21_DCV_V06/GWM/Battery_Traction_4_FD1 ==
  BattTracDiagClr_B_Rq : Constant
  BattTracSoc2_Pc_Actl : Constant
  BattTrac_Te_Actl : Constant
  bus_creator : BusCreator  Inputs=3
  port : Outport
  wires:
  bus_creator/1 -> port/1  "Battery_Traction_4_FD1"
  BattTracDiagClr_B_Rq/1 -> bus_creator/1  "BattTracDiagClr_B_Rq"
  BattTracSoc2_Pc_Actl/1 -> bus_creator/2  "BattTracSoc2_Pc_Actl"
  BattTrac_Te_Actl/1 -> bus_creator/3  "BattTrac_Te_Actl"

== system test_mdl/FD1_CAN_P702_GASD_MY21_DCV_V06/GWM/Battery_Traction_5_FD1 ==
  BattTrac2_Pw_ChrgInst : Constant
  BattTrac2_Pw_DchrgInst : Constant
  BattTrac2_Pw_LimChrg : Constant
  BattTrac2_Pw_LimDchrg : Constant
  bus_creator : BusCreator  Inputs=4
  port : Outport
  wires:
  bus_creator/1 -> port/1  "Battery_Traction_5_FD1"
  BattTrac2_Pw_ChrgInst/1 -> bus_creator/1  "BattTrac2_Pw_ChrgInst"
  BattTrac2_Pw_DchrgInst/1 -> bus_creator/2  "BattTrac2_Pw_DchrgInst"
  BattTrac2_Pw_LimChrg/1 -> bus_creator/3  "BattTrac2_Pw_LimChrg"
  BattTrac2_Pw_LimDchrg/1 -> bus_creator/4  "BattTrac2_Pw_LimDchrg"

== system test_mdl/FD1_CAN_P702_GASD_MY21_DCV_V06/GWM/Battery_Traction_6_FD1 ==
  BattTracChrgSustn_B_Rq : Constant
  BattTracClntPmp_D_Stat : Constant
  BattTracCnnct_D_Cmd : Constant
  BattTracDcdcDis_B_Rq : Constant
  BattTracDelta_Te_Actl : Constant
  BattTracHvilOpen_B_Stat : Constant
  HtrnClntPump_D_Stat : Constant
  bus_creator : BusCreator  Inputs=7
  port : Outport
  wires:
  bus_creator/1 -> port/1  "Battery_Traction_6_FD1"
  BattTracChrgSustn_B_Rq/1 -> bus_creator/1  "BattTracChrgSustn_B_Rq"
  BattTracClntPmp_D_Stat/1 -> bus_creator/2  "BattTracClntPmp_D_Stat"
  BattTracCnnct_D_Cmd/1 -> bus_creator/3  "BattTracCnnct_D_Cmd"
  BattTracDcdcDis_B_Rq/1 -> bus_creator/4  "BattTracDcdcDis_B_Rq"
  BattTracDelta_Te_Actl/1 -> bus_creator/5  "BattTracDelta_Te_Actl"
  BattTracHvilOpen_B_Stat/1 -> bus_creator/6  "BattTracHvilOpen_B_Stat"
  HtrnClntPump_D_Stat/1 -> bus_creator/7  "HtrnClntPump_D_Stat"

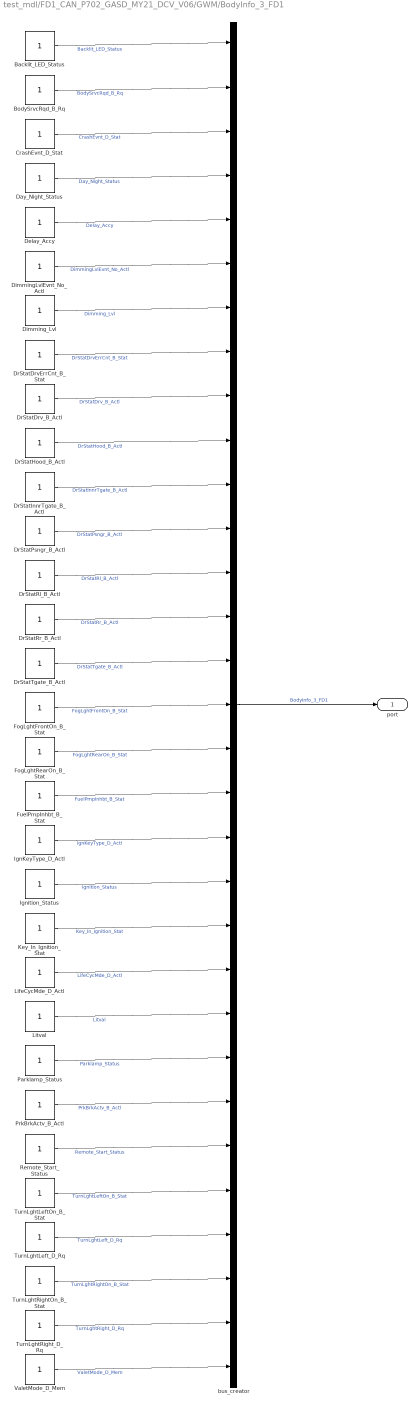
== system test_mdl/FD1_CAN_P702_GASD_MY21_DCV_V06/GWM/BodyInfo_3_FD1 ==
  Backlit_LED_Status : Constant
  BodySrvcRqd_B_Rq : Constant
  CrashEvnt_D_Stat : Constant
  Day_Night_Status : Constant
  Delay_Accy : Constant
  DimmingLvlEvnt_No_Actl : Constant
  Dimming_Lvl : Constant
  DrStatDrvErrCnt_B_Stat : Constant
  DrStatDrv_B_Actl : Constant
  DrStatHood_B_Actl : Constant
  DrStatInnrTgate_B_Actl : Constant
  DrStatPsngr_B_Actl : Constant
  DrStatRl_B_Actl : Constant
  DrStatRr_B_Actl : Constant
  DrStatTgate_B_Actl : Constant
  FogLghtFrontOn_B_Stat : Constant
  FogLghtRearOn_B_Stat : Constant
  FuelPmpInhbt_B_Stat : Constant
  IgnKeyType_D_Actl : Constant
  Ignition_Status : Constant
  Key_In_Ignition_Stat : Constant
  LifeCycMde_D_Actl : Constant
  Litval : Constant
  Parklamp_Status : Constant
  PrkBrkActv_B_Actl : Constant
  Remote_Start_Status : Constant
  TurnLghtLeftOn_B_Stat : Constant
  TurnLghtLeft_D_Rq : Constant
  TurnLghtRightOn_B_Stat : Constant
  TurnLghtRight_D_Rq : Constant
  ValetMode_D_Mem : Constant
  bus_creator : BusCreator  Inputs=31
  port : Outport
  wires:
  bus_creator/1 -> port/1  "BodyInfo_3_FD1"
  Backlit_LED_Status/1 -> bus_creator/1  "Backlit_LED_Status"
  BodySrvcRqd_B_Rq/1 -> bus_creator/2  "BodySrvcRqd_B_Rq"
  CrashEvnt_D_Stat/1 -> bus_creator/3  "CrashEvnt_D_Stat"
  Day_Night_Status/1 -> bus_creator/4  "Day_Night_Status"
  Delay_Accy/1 -> bus_creator/5  "Delay_Accy"
  DimmingLvlEvnt_No_Actl/1 -> bus_creator/6  "DimmingLvlEvnt_No_Actl"
  Dimming_Lvl/1 -> bus_creator/7  "Dimming_Lvl"
  DrStatDrvErrCnt_B_Stat/1 -> bus_creator/8  "DrStatDrvErrCnt_B_Stat"
  DrStatDrv_B_Actl/1 -> bus_creator/9  "DrStatDrv_B_Actl"
  DrStatHood_B_Actl/1 -> bus_creator/10  "DrStatHood_B_Actl"
  DrStatInnrTgate_B_Actl/1 -> bus_creator/11  "DrStatInnrTgate_B_Actl"
  DrStatPsngr_B_Actl/1 -> bus_creator/12  "DrStatPsngr_B_Actl"
  DrStatRl_B_Actl/1 -> bus_creator/13  "DrStatRl_B_Actl"
  DrStatRr_B_Actl/1 -> bus_creator/14  "DrStatRr_B_Actl"
  DrStatTgate_B_Actl/1 -> bus_creator/15  "DrStatTgate_B_Actl"
  FogLghtFrontOn_B_Stat/1 -> bus_creator/16  "FogLghtFrontOn_B_Stat"
  FogLghtRearOn_B_Stat/1 -> bus_creator/17  "FogLghtRearOn_B_Stat"
  FuelPmpInhbt_B_Stat/1 -> bus_creator/18  "FuelPmpInhbt_B_Stat"
  IgnKeyType_D_Actl/1 -> bus_creator/19  "IgnKeyType_D_Actl"
  Ignition_Status/1 -> bus_creator/20  "Ignition_Status"
  Key_In_Ignition_Stat/1 -> bus_creator/21  "Key_In_Ignition_Stat"
  LifeCycMde_D_Actl/1 -> bus_creator/22  "LifeCycMde_D_Actl"
  Litval/1 -> bus_creator/23  "Litval"
  Parklamp_Status/1 -> bus_creator/24  "Parklamp_Status"
  PrkBrkActv_B_Actl/1 -> bus_creator/25  "PrkBrkActv_B_Actl"
  Remote_Start_Status/1 -> bus_creator/26  "Remote_Start_Status"
  TurnLghtLeftOn_B_Stat/1 -> bus_creator/27  "TurnLghtLeftOn_B_Stat"
  TurnLghtLeft_D_Rq/1 -> bus_creator/28  "TurnLghtLeft_D_Rq"
  TurnLghtRightOn_B_Stat/1 -> bus_creator/29  "TurnLghtRightOn_B_Stat"
  TurnLghtRight_D_Rq/1 -> bus_creator/30  "TurnLghtRight_D_Rq"
  ValetMode_D_Mem/1 -> bus_creator/31  "ValetMode_D_Mem"

== system test_mdl/FD1_CAN_P702_GASD_MY21_DCV_V06/GWM/Body_Info_10_FD1 ==
  GenericSwtch1_No_Actl : Constant
  GenericSwtch2_No_Actl : Constant
  GenericSwtch3_No_Actl : Constant
  bus_creator : BusCreator  Inputs=3
  port : Outport
  wires:
  bus_creator/1 -> port/1  "Body_Info_10_FD1"
  GenericSwtch1_No_Actl/1 -> bus_creator/1  "GenericSwtch1_No_Actl"
  GenericSwtch2_No_Actl/1 -> bus_creator/2  "GenericSwtch2_No_Actl"
  GenericSwtch3_No_Actl/1 -> bus_creator/3  "GenericSwtch3_No_Actl"

== system test_mdl/FD1_CAN_P702_GASD_MY21_DCV_V06/GWM/Body_Info_4_FD1 ==
  BattULo_I_Actl : Constant
  BattULo_U_Actl : Constant
  BrkTrnShifLck_B_Stat : Constant
  DcacElPw_D_Rq : Constant
  DriverCrankingReq : Constant
  EngOff_T_Actl : Constant
  FuelPumpPwr_D_Stat : Constant
  PrkLckCtlAvail_T_Stat : Constant
  PrkLckCtlMsgTxt_D_Rq : Constant
  PrkLckCtlTow_B_Enbl : Constant
  PrkLckCtlUnlck_D_Stat : Constant
  PrkLckCtl_B_Enbl : Constant
  PtLatchActv_B_RqBcm : Constant
  ReFuelSwtchStat_D_Actl : Constant
  bus_creator : BusCreator  Inputs=15
  immoSecureIdleMode : Constant
  port : Outport
  wires:
  bus_creator/1 -> port/1  "Body_Info_4_FD1"
  BattULo_I_Actl/1 -> bus_creator/1  "BattULo_I_Actl"
  BattULo_U_Actl/1 -> bus_creator/2  "BattULo_U_Actl"
  BrkTrnShifLck_B_Stat/1 -> bus_creator/3  "BrkTrnShifLck_B_Stat"
  DcacElPw_D_Rq/1 -> bus_creator/4  "DcacElPw_D_Rq"
  DriverCrankingReq/1 -> bus_creator/5  "DriverCrankingReq"
  EngOff_T_Actl/1 -> bus_creator/6  "EngOff_T_Actl"
  FuelPumpPwr_D_Stat/1 -> bus_creator/7  "FuelPumpPwr_D_Stat"
  PrkLckCtlAvail_T_Stat/1 -> bus_creator/8  "PrkLckCtlAvail_T_Stat"
  PrkLckCtlMsgTxt_D_Rq/1 -> bus_creator/9  "PrkLckCtlMsgTxt_D_Rq"
  PrkLckCtlTow_B_Enbl/1 -> bus_creator/10  "PrkLckCtlTow_B_Enbl"
  PrkLckCtlUnlck_D_Stat/1 -> bus_creator/11  "PrkLckCtlUnlck_D_Stat"
  PrkLckCtl_B_Enbl/1 -> bus_creator/12  "PrkLckCtl_B_Enbl"
  PtLatchActv_B_RqBcm/1 -> bus_creator/13  "PtLatchActv_B_RqBcm"
  ReFuelSwtchStat_D_Actl/1 -> bus_creator/14  "ReFuelSwtchStat_D_Actl"
  immoSecureIdleMode/1 -> bus_creator/15  "immoSecureIdleMode"

== system test_mdl/FD1_CAN_P702_GASD_MY21_DCV_V06/GWM/Body_Info_6_FD1 ==
  DrLatchMsgTxt_D_Rq : Constant
  ElPwPoint_D_Rq : Constant
  HeadLghtHiPrmsn_D_Stat : Constant
  IgnPsswrdDsply_B_Rq : Constant
  KeyAdmnTot_No_Cnt : Constant
  KeyMykeyTot_No_Cnt : Constant
  Keycode_Status : Constant
  PEBackupSlot_Stats : Constant
  PoliceIdlMde_D_Stat : Constant
  PrmtrAlrmEvnt_D_Stat : Constant
  PrsnlDevcChrgEnbl_B_Rq : Constant
  SecurityMsgTxt_D_Rq : Constant
  SteWhlLckMsgTxt_D_Rq : Constant
  TracKeyMde_D_Stat : Constant
  bus_creator : BusCreator  Inputs=15
  immoMsgTxt_D_Rq : Constant
  port : Outport
  wires:
  bus_creator/1 -> port/1  "Body_Info_6_FD1"
  DrLatchMsgTxt_D_Rq/1 -> bus_creator/1  "DrLatchMsgTxt_D_Rq"
  ElPwPoint_D_Rq/1 -> bus_creator/2  "ElPwPoint_D_Rq"
  HeadLghtHiPrmsn_D_Stat/1 -> bus_creator/3  "HeadLghtHiPrmsn_D_Stat"
  IgnPsswrdDsply_B_Rq/1 -> bus_creator/4  "IgnPsswrdDsply_B_Rq"
  KeyAdmnTot_No_Cnt/1 -> bus_creator/5  "KeyAdmnTot_No_Cnt"
  KeyMykeyTot_No_Cnt/1 -> bus_creator/6  "KeyMykeyTot_No_Cnt"
  Keycode_Status/1 -> bus_creator/7  "Keycode_Status"
  PEBackupSlot_Stats/1 -> bus_creator/8  "PEBackupSlot_Stats"
  PoliceIdlMde_D_Stat/1 -> bus_creator/9  "PoliceIdlMde_D_Stat"
  PrmtrAlrmEvnt_D_Stat/1 -> bus_creator/10  "PrmtrAlrmEvnt_D_Stat"
  PrsnlDevcChrgEnbl_B_Rq/1 -> bus_creator/11  "PrsnlDevcChrgEnbl_B_Rq"
  SecurityMsgTxt_D_Rq/1 -> bus_creator/12  "SecurityMsgTxt_D_Rq"
  SteWhlLckMsgTxt_D_Rq/1 -> bus_creator/13  "SteWhlLckMsgTxt_D_Rq"
  TracKeyMde_D_Stat/1 -> bus_creator/14  "TracKeyMde_D_Stat"
  immoMsgTxt_D_Rq/1 -> bus_creator/15  "immoMsgTxt_D_Rq"

== system test_mdl/FD1_CAN_P702_GASD_MY21_DCV_V06/GWM/Body_Info_8_FD1 ==
  BattRgenLoChrg_D_Rq : Constant
  BattRgenLoDChrg_D_Rq : Constant
  ChrgCordLck_B_Stat : Constant
  ChrgCordResp1_No_Actl : Constant
  ChrgCordResp2_No_Actl : Constant
  WakeAlarm0_D_Stat : Constant
  WakeAlarm1_D_Stat : Constant
  WakeAlarm2_D_Stat : Constant
  WakeAlarm3_D_Stat : Constant
  bus_creator : BusCreator  Inputs=9
  port : Outport
  wires:
  bus_creator/1 -> port/1  "Body_Info_8_FD1"
  BattRgenLoChrg_D_Rq/1 -> bus_creator/1  "BattRgenLoChrg_D_Rq"
  BattRgenLoDChrg_D_Rq/1 -> bus_creator/2  "BattRgenLoDChrg_D_Rq"
  ChrgCordLck_B_Stat/1 -> bus_creator/3  "ChrgCordLck_B_Stat"
  ChrgCordResp1_No_Actl/1 -> bus_creator/4  "ChrgCordResp1_No_Actl"
  ChrgCordResp2_No_Actl/1 -> bus_creator/5  "ChrgCordResp2_No_Actl"
  WakeAlarm0_D_Stat/1 -> bus_creator/6  "WakeAlarm0_D_Stat"
  WakeAlarm1_D_Stat/1 -> bus_creator/7  "WakeAlarm1_D_Stat"
  WakeAlarm2_D_Stat/1 -> bus_creator/8  "WakeAlarm2_D_Stat"
  WakeAlarm3_D_Stat/1 -> bus_creator/9  "WakeAlarm3_D_Stat"

== system test_mdl/FD1_CAN_P702_GASD_MY21_DCV_V06/GWM/Body_Info_9_FD1 ==
  AdvStrt_D_Stat : Constant
  CrnkInhbt_B_Stat : Constant
  CrnkInhbt_No_Cnt : Constant
  CrnkInhbt_No_Cs : Constant
  DrvInCtl_B_Stat : Constant
  EngStrtActv_B_Stat : Constant
  EngStrt_B_Rq : Constant
  IgnPreOffActv_B_Stat : Constant
  PtWakeReas_D_Stat : Constant
  StrtrMtrCtlDStat_No_Cs : Constant
  VehOnSrc_D_Stat : Constant
  bus_creator : BusCreator  Inputs=11
  port : Outport
  wires:
  bus_creator/1 -> port/1  "Body_Info_9_FD1"
  AdvStrt_D_Stat/1 -> bus_creator/1  "AdvStrt_D_Stat"
  CrnkInhbt_B_Stat/1 -> bus_creator/2  "CrnkInhbt_B_Stat"
  CrnkInhbt_No_Cnt/1 -> bus_creator/3  "CrnkInhbt_No_Cnt"
  CrnkInhbt_No_Cs/1 -> bus_creator/4  "CrnkInhbt_No_Cs"
  DrvInCtl_B_Stat/1 -> bus_creator/5  "DrvInCtl_B_Stat"
  EngStrtActv_B_Stat/1 -> bus_creator/6  "EngStrtActv_B_Stat"
  EngStrt_B_Rq/1 -> bus_creator/7  "EngStrt_B_Rq"
  IgnPreOffActv_B_Stat/1 -> bus_creator/8  "IgnPreOffActv_B_Stat"
  PtWakeReas_D_Stat/1 -> bus_creator/9  "PtWakeReas_D_Stat"
  StrtrMtrCtlDStat_No_Cs/1 -> bus_creator/10  "StrtrMtrCtlDStat_No_Cs"
  VehOnSrc_D_Stat/1 -> bus_creator/11  "VehOnSrc_D_Stat"

== system test_mdl/FD1_CAN_P702_GASD_MY21_DCV_V06/GWM/Climate_Cntrl_Data_2_FD1 ==
  AutoStpHvacDelta_I_Est : Constant
  CabnAmb_Te_Actl : Constant
  ClimtThrmlLoad_No_Actl : Constant
  HvacAir_Flw_Est : Constant
  HvacBlwrFront_D_Stat : Constant
  HvacRec_Pc_Est : Constant
  HvacRemoteStrt_N_Rq : Constant
  bus_creator : BusCreator  Inputs=7
  port : Outport
  wires:
  bus_creator/1 -> port/1  "Climate_Cntrl_Data_2_FD1"
  AutoStpHvacDelta_I_Est/1 -> bus_creator/1  "AutoStpHvacDelta_I_Est"
  CabnAmb_Te_Actl/1 -> bus_creator/2  "CabnAmb_Te_Actl"
  ClimtThrmlLoad_No_Actl/1 -> bus_creator/3  "ClimtThrmlLoad_No_Actl"
  HvacAir_Flw_Est/1 -> bus_creator/4  "HvacAir_Flw_Est"
  HvacBlwrFront_D_Stat/1 -> bus_creator/5  "HvacBlwrFront_D_Stat"
  HvacRec_Pc_Est/1 -> bus_creator/6  "HvacRec_Pc_Est"
  HvacRemoteStrt_N_Rq/1 -> bus_creator/7  "HvacRemoteStrt_N_Rq"

== system test_mdl/FD1_CAN_P702_GASD_MY21_DCV_V06/GWM/Climate_Control_Data_FD1 ==
  AutoHoldSwtch_D_Stat : Constant
  LpdbDfrstRearOn_B_Rq : Constant
  LpdbHeatWiprPrk_B_Rq : Constant
  LpdbPtc1_B_Rq : Constant
  LpdbPtc2_B_Rq : Constant
  LpdbPtc3_B_Rq : Constant
  MirrorHeatOn_B_Rq : Constant
  Outside_Air_Temp_Stat : Constant
  Remote_Start_QuietMode : Constant
  SteWhlHeat_D_Rq : Constant
  bus_creator : BusCreator  Inputs=10
  port : Outport
  wires:
  bus_creator/1 -> port/1  "Climate_Control_Data_FD1"
  AutoHoldSwtch_D_Stat/1 -> bus_creator/1  "AutoHoldSwtch_D_Stat"
  LpdbDfrstRearOn_B_Rq/1 -> bus_creator/2  "LpdbDfrstRearOn_B_Rq"
  LpdbHeatWiprPrk_B_Rq/1 -> bus_creator/3  "LpdbHeatWiprPrk_B_Rq"
  LpdbPtc1_B_Rq/1 -> bus_creator/4  "LpdbPtc1_B_Rq"
  LpdbPtc2_B_Rq/1 -> bus_creator/5  "LpdbPtc2_B_Rq"
  LpdbPtc3_B_Rq/1 -> bus_creator/6  "LpdbPtc3_B_Rq"
  MirrorHeatOn_B_Rq/1 -> bus_creator/7  "MirrorHeatOn_B_Rq"
  Outside_Air_Temp_Stat/1 -> bus_creator/8  "Outside_Air_Temp_Stat"
  Remote_Start_QuietMode/1 -> bus_creator/9  "Remote_Start_QuietMode"
  SteWhlHeat_D_Rq/1 -> bus_creator/10  "SteWhlHeat_D_Rq"

== system test_mdl/FD1_CAN_P702_GASD_MY21_DCV_V06/GWM/Cluster_HEV_Data8_FD1 ==
  ConsAvgTrip_Fe_Dsply : Constant
  DrvEffLvl_No_Stat : Constant
  EngAirFilt_B_RqReset : Constant
  GpsElMdeSel_B_Rq : Constant
  LongTermReset_B_Rq : Constant
  bus_creator : BusCreator  Inputs=5
  port : Outport
  wires:
  bus_creator/1 -> port/1  "Cluster_HEV_Data8_FD1"
  ConsAvgTrip_Fe_Dsply/1 -> bus_creator/1  "ConsAvgTrip_Fe_Dsply"
  DrvEffLvl_No_Stat/1 -> bus_creator/2  "DrvEffLvl_No_Stat"
  EngAirFilt_B_RqReset/1 -> bus_creator/3  "EngAirFilt_B_RqReset"
  GpsElMdeSel_B_Rq/1 -> bus_creator/4  "GpsElMdeSel_B_Rq"
  LongTermReset_B_Rq/1 -> bus_creator/5  "LongTermReset_B_Rq"

== system test_mdl/FD1_CAN_P702_GASD_MY21_DCV_V06/GWM/Cluster_Info1_FD1 ==
  AccDeny_B_RqIpc : Constant
  AccEnbl_B_RqDrv : Constant
  BulbChkActv_B_Stat : Constant
  DrvSlipCtlMde_B_Rq2 : Constant
  DrvSlipCtlMde_D_Rq : Constant
  EngIdlShutDown_B_RqDrv : Constant
  EngOilLife_B_RqReset : Constant
  HaDsplyCpblty_B_Stat : Constant
  HsaMde_D_Rq : Constant
  KeyTypeChngMykey_D_Rq : Constant
  LscmbbStat_B_Actl : Constant
  ManRgen_D_Rq : Constant
  MetricActv_B_Actl : Constant
  NtrlTowMdeEnbl_B_RqDrv : Constant
  OdometerMasterValue : Constant
  ParkDetect_Stat : Constant
  Power_Liftgate_Mode_Cmd : Constant
  ReducedGuard_D_Rq : Constant
  TRAILER_BRAKE_CONFIG : Constant
  TRLR_SWAY_CONFIG_CMD : Constant
  TrlrBrkMde_D_Rq : Constant
  bus_creator : BusCreator  Inputs=22
  ePRNDL_MODE : Constant
  port : Outport
  wires:
  bus_creator/1 -> port/1  "Cluster_Info1_FD1"
  AccDeny_B_RqIpc/1 -> bus_creator/1  "AccDeny_B_RqIpc"
  AccEnbl_B_RqDrv/1 -> bus_creator/2  "AccEnbl_B_RqDrv"
  BulbChkActv_B_Stat/1 -> bus_creator/3  "BulbChkActv_B_Stat"
  DrvSlipCtlMde_B_Rq2/1 -> bus_creator/4  "DrvSlipCtlMde_B_Rq2"
  DrvSlipCtlMde_D_Rq/1 -> bus_creator/5  "DrvSlipCtlMde_D_Rq"
  EngIdlShutDown_B_RqDrv/1 -> bus_creator/6  "EngIdlShutDown_B_RqDrv"
  EngOilLife_B_RqReset/1 -> bus_creator/7  "EngOilLife_B_RqReset"
  HaDsplyCpblty_B_Stat/1 -> bus_creator/8  "HaDsplyCpblty_B_Stat"
  HsaMde_D_Rq/1 -> bus_creator/9  "HsaMde_D_Rq"
  KeyTypeChngMykey_D_Rq/1 -> bus_creator/10  "KeyTypeChngMykey_D_Rq"
  LscmbbStat_B_Actl/1 -> bus_creator/11  "LscmbbStat_B_Actl"
  ManRgen_D_Rq/1 -> bus_creator/12  "ManRgen_D_Rq"
  MetricActv_B_Actl/1 -> bus_creator/13  "MetricActv_B_Actl"
  NtrlTowMdeEnbl_B_RqDrv/1 -> bus_creator/14  "NtrlTowMdeEnbl_B_RqDrv"
  OdometerMasterValue/1 -> bus_creator/15  "OdometerMasterValue"
  ParkDetect_Stat/1 -> bus_creator/16  "ParkDetect_Stat"
  Power_Liftgate_Mode_Cmd/1 -> bus_creator/17  "Power_Liftgate_Mode_Cmd"
  ReducedGuard_D_Rq/1 -> bus_creator/18  "ReducedGuard_D_Rq"
  TRAILER_BRAKE_CONFIG/1 -> bus_creator/19  "TRAILER_BRAKE_CONFIG"
  TRLR_SWAY_CONFIG_CMD/1 -> bus_creator/20  "TRLR_SWAY_CONFIG_CMD"
  TrlrBrkMde_D_Rq/1 -> bus_creator/21  "TrlrBrkMde_D_Rq"
  ePRNDL_MODE/1 -> bus_creator/22  "ePRNDL_MODE"

== system test_mdl/FD1_CAN_P702_GASD_MY21_DCV_V06/GWM/Cluster_Info_3_FD1 ==
  AutoRgen_D_Rq : Constant
  DISPLAY_SPEED_OFFSET : Constant
  DISPLAY_SPEED_SCALING : Constant
  DrvSlipCtlMde_B_RqMyKey : Constant
  FUEL_SENSOR_NUM : Constant
  FuelLvlActvSide_No_Raw : Constant
  FuelLvlPssvSide_No_Raw : Constant
  FuelLvlWarn_D_Actl : Constant
  FuelLvl_Pc_Dsply : Constant
  FuelSecndActv_B_Actl : Constant
  HILL_DESC_SW : Constant
  OdoTripRx_B_Actl : Constant
  Veh_V_CompLimMx : Constant
  W2S_LAMP_OK : Constant
  bus_creator : BusCreator  Inputs=14
  port : Outport
  wires:
  bus_creator/1 -> port/1  "Cluster_Info_3_FD1"
  AutoRgen_D_Rq/1 -> bus_creator/1  "AutoRgen_D_Rq"
  DISPLAY_SPEED_OFFSET/1 -> bus_creator/2  "DISPLAY_SPEED_OFFSET"
  DISPLAY_SPEED_SCALING/1 -> bus_creator/3  "DISPLAY_SPEED_SCALING"
  DrvSlipCtlMde_B_RqMyKey/1 -> bus_creator/4  "DrvSlipCtlMde_B_RqMyKey"
  FUEL_SENSOR_NUM/1 -> bus_creator/5  "FUEL_SENSOR_NUM"
  FuelLvlActvSide_No_Raw/1 -> bus_creator/6  "FuelLvlActvSide_No_Raw"
  FuelLvlPssvSide_No_Raw/1 -> bus_creator/7  "FuelLvlPssvSide_No_Raw"
  FuelLvlWarn_D_Actl/1 -> bus_creator/8  "FuelLvlWarn_D_Actl"
  FuelLvl_Pc_Dsply/1 -> bus_creator/9  "FuelLvl_Pc_Dsply"
  FuelSecndActv_B_Actl/1 -> bus_creator/10  "FuelSecndActv_B_Actl"
  HILL_DESC_SW/1 -> bus_creator/11  "HILL_DESC_SW"
  OdoTripRx_B_Actl/1 -> bus_creator/12  "OdoTripRx_B_Actl"
  Veh_V_CompLimMx/1 -> bus_creator/13  "Veh_V_CompLimMx"
  W2S_LAMP_OK/1 -> bus_creator/14  "W2S_LAMP_OK"

== system test_mdl/FD1_CAN_P702_GASD_MY21_DCV_V06/GWM/Cluster_Lighting_Rq_FD1 ==
  IsaOffst_D_Rq : Constant
  SlMde_D_Rq : Constant
  bus_creator : BusCreator  Inputs=2
  port : Outport
  wires:
  bus_creator/1 -> port/1  "Cluster_Lighting_Rq_FD1"
  IsaOffst_D_Rq/1 -> bus_creator/1  "IsaOffst_D_Rq"
  SlMde_D_Rq/1 -> bus_creator/2  "SlMde_D_Rq"

== system test_mdl/FD1_CAN_P702_GASD_MY21_DCV_V06/GWM/Compressor_Req_FD1 ==
  ClimtCool_D_Rq : Constant
  ClimtHeat_D_Rq : Constant
  ClimtPw_B_Rq : Constant
  HvacAirCond_B_Rq : Constant
  HvacEvap_Te_Actl : Constant
  HvacEvap_Te_Offst : Constant
  HvacEvap_Te_Rq : Constant
  HvacHtrCore_Te_Rq : Constant
  SnowPlowMde_B_Enbl : Constant
  StopStrtDrvMde_B_RqBtn : Constant
  bus_creator : BusCreator  Inputs=10
  port : Outport
  wires:
  bus_creator/1 -> port/1  "Compressor_Req_FD1"
  ClimtCool_D_Rq/1 -> bus_creator/1  "ClimtCool_D_Rq"
  ClimtHeat_D_Rq/1 -> bus_creator/2  "ClimtHeat_D_Rq"
  ClimtPw_B_Rq/1 -> bus_creator/3  "ClimtPw_B_Rq"
  HvacAirCond_B_Rq/1 -> bus_creator/4  "HvacAirCond_B_Rq"
  HvacEvap_Te_Actl/1 -> bus_creator/5  "HvacEvap_Te_Actl"
  HvacEvap_Te_Offst/1 -> bus_creator/6  "HvacEvap_Te_Offst"
  HvacEvap_Te_Rq/1 -> bus_creator/7  "HvacEvap_Te_Rq"
  HvacHtrCore_Te_Rq/1 -> bus_creator/8  "HvacHtrCore_Te_Rq"
  SnowPlowMde_B_Enbl/1 -> bus_creator/9  "SnowPlowMde_B_Enbl"
  StopStrtDrvMde_B_RqBtn/1 -> bus_creator/10  "StopStrtDrvMde_B_RqBtn"
